simulink model "AGSTSMO"  (R2021a)
settings: Solver=ode113  StartTime=0.0  StopTime=10  FixedStep=10e-4  RelTol=1e-5
settings Model: Creator=LENOVO PC  LastModifiedBy=Dell
settings SolverCC: AlgebraicLoopSolver=TrustRegion
settings DataIOCC: ReturnWorkspaceOutputs=off
settings DebuggingCC: SFMachineParentedDataDiag=warning

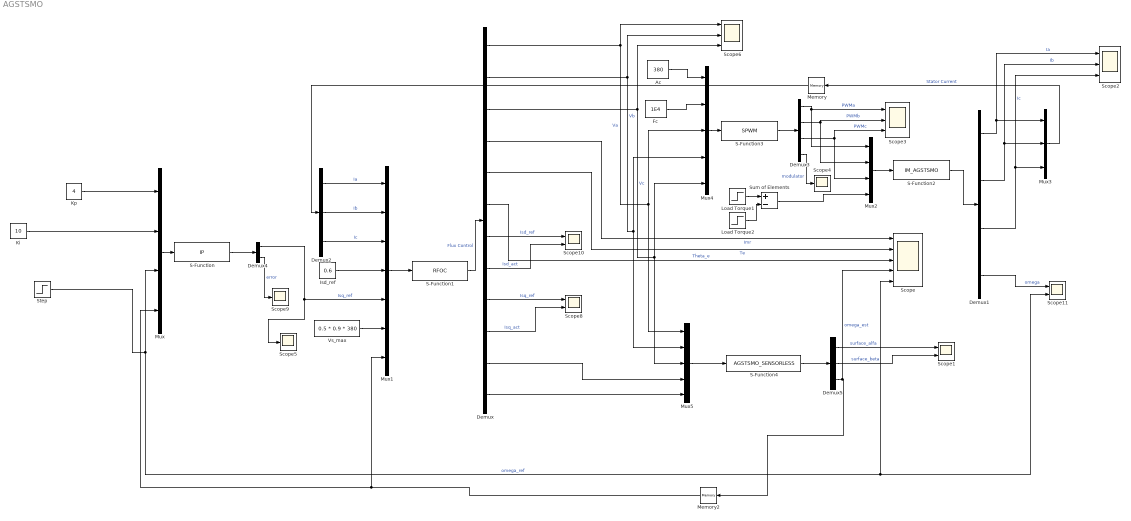
== system AGSTSMO ==
  Ac : Constant  Value=380
  Demux : Demux  Outputs=12
  Demux1 : Demux
  Demux2 : Demux  Outputs=3
  Demux3 : Demux
  Demux4 : Demux  Outputs=2
  Demux5 : Demux  Outputs=3
  Fc : Constant  Value=1E4
  Isd_ref : Constant  Value=0.6
  Ki : Constant  Value=10
  Kp : Constant  Value=4
  Load Torque1 : Step  Time=3  After=3  SampleTime=0
  Load Torque2 : Step  Time=7  After=3  SampleTime=0
  Memory : Memory
  Memory2 : Memory
  Mux : Mux
  Mux1 : Mux  Inputs=7
  Mux2 : Mux
  Mux3 : Mux  Inputs=3
  Mux4 : Mux  Inputs=5
  Mux5 : Mux  Inputs=5
  S-Function : S-Function  FunctionName=IP  SFunctionDeploymentMode=off  EnableBusSupport=off
  S-Function1 : S-Function  FunctionName=RFOC  SFunctionDeploymentMode=off  EnableBusSupport=off
  S-Function2 : S-Function  FunctionName=IM_AGSTSMO  SFunctionDeploymentMode=off  EnableBusSupport=off
  S-Function3 : S-Function  FunctionName=SPWM  SFunctionDeploymentMode=off  EnableBusSupport=off
  S-Function4 : S-Function  FunctionName=AGSTSMO_SENSORLESS  SFunctionDeploymentMode=off  EnableBusSupport=off
  Scope : Scope  NumInputPorts=5
  Scope{1,8,10..11} (4 alike) : Scope  NumInputPorts=2
  Scope2 : Scope  NumInputPorts=3
  Scope3 : Scope  NumInputPorts=3
  Scope4 : Scope
  Scope5 : Scope
  Scope6 : Scope  NumInputPorts=3
  Scope9 : Scope
  Step : Step  Time=0  After=10  SampleTime=0
  Sum of Elements : Sum  Inputs=+-
  Vs_max : Constant  Value=0.5 * 0.9 * 380
  wires:
  Mux/1 -> S-Function/1
  Ki/1 -> Mux/2
  Memory2/1 -> Mux1/7, Mux/4
  Memory/1 -> Demux2/1
  Mux2/1 -> S-Function2/1
  Demux1/3 -> Scope2/3, Mux3/3  "Ic"
  Ac/1 -> Mux4/1
  Demux2/1 -> Mux1/1  "Ia"
  Demux2/2 -> Mux1/2  "Ib"
  Mux3/1 -> Memory/1  "Stator Current"
  Demux1/2 -> Scope2/2, Mux3/2  "Ib"
  S-Function2/1 -> Demux1/1
  Kp/1 -> Mux/1
  Demux1/1 -> Mux3/1, Scope2/1  "Ia"
  Demux2/3 -> Mux1/3  "Ic"
  S-Function1/1 -> Demux/1  "Flux Control"
  Mux1/1 -> S-Function1/1
  Fc/1 -> Mux4/2
  Demux3/1 -> Mux2/1, Scope3/1  "PWMa"
  Demux3/2 -> Scope3/2, Mux2/2  "PWMb"
  Demux3/3 -> Scope3/3, Mux2/3  "PWMc"
  Demux3/4 -> Scope4/1  "modulator"
  Isd_ref/1 -> Mux1/4
  Demux/1 -> Mux4/3, Mux5/1, Scope6/1  "Va"
  Demux/2 -> Mux4/4, Mux5/2, Scope6/2  "Vb"
  Demux/3 -> Mux5/3, Mux4/5, Scope6/3  "Vc"
  S-Function/1 -> Demux4/1
  Demux4/1 -> Mux1/5, Scope5/1  "Isq_ref"
  Demux4/2 -> Scope9/1  "error"
  Step/1 -> Scope/5, Scope11/2, Mux/3  "omega_ref"
  Demux1/4 -> Scope11/1  "omega"
  Vs_max/1 -> Mux1/6
  Mux4/1 -> S-Function3/1
  S-Function3/1 -> Demux3/1
  Mux5/1 -> S-Function4/1
  S-Function4/1 -> Demux5/1
  Demux5/1 -> Scope1/1  "surface_alfa"
  Demux5/2 -> Scope1/2  "surface_beta"
  Demux5/3 -> Scope/4, Memory2/1  "omega_est"
  Demux/11 -> Mux5/4
  Demux/12 -> Mux5/5
  Demux/4 -> Scope/1  "Imr"
  Demux/5 -> Scope/2  "Te"
  Demux/6 -> Scope/3  "Theta_e"
  Demux/7 -> Scope10/1  "Isd_ref"
  Demux/8 -> Scope10/2  "Isd_act"
  Demux/9 -> Scope8/1  "Isq_ref"
  Demux/10 -> Scope8/2  "Isq_act"
  Load Torque1/1 -> Sum of Elements/1
  Load Torque2/1 -> Sum of Elements/2
  Sum of Elements/1 -> Mux2/4
